simulink model "tf_scope"  (R2023b)
settings: Solver=VariableStepAuto  StartTime=0.0  StopTime=10.0  RelTol=1e-3
settings Model: Creator=monica  LastModifiedBy=monica

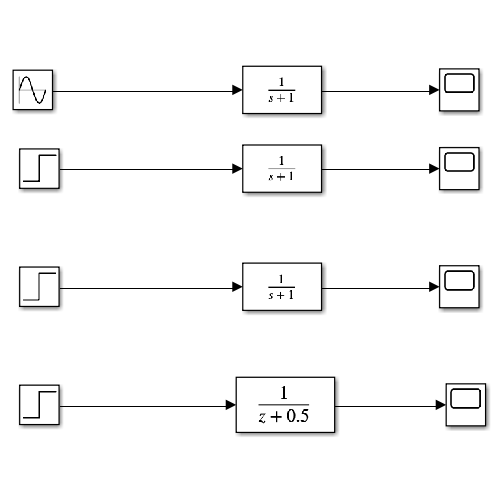
[thumbnail: Simulink's stored preview of the top-level diagram]
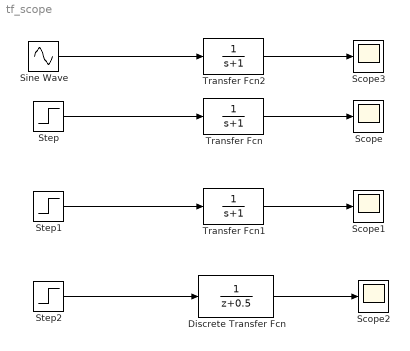
== system tf_scope ==
  Discrete Transfer Fcn : DiscreteTransferFcn
  Scope{,1..3} (4 alike) : Scope
  Sine Wave : Sin  SampleTime=0
  Step : Step  SampleTime=0
  Step1 : Step  SampleTime=0
  Step2 : Step  SampleTime=0
  Transfer Fcn : TransferFcn  Denominator=[1 1]
  Transfer Fcn1 : TransferFcn  Denominator=[1 1]
  Transfer Fcn2 : TransferFcn  Denominator=[1 1]
  wires:
  Step/1 -> Transfer Fcn/1
  Transfer Fcn/1 -> Scope/1
  Step1/1 -> Transfer Fcn1/1
  Transfer Fcn1/1 -> Scope1/1
  Step2/1 -> Discrete Transfer Fcn/1
  Discrete Transfer Fcn/1 -> Scope2/1
  Sine Wave/1 -> Transfer Fcn2/1
  Transfer Fcn2/1 -> Scope3/1
